simulink model "cruise_control"  (R2020b)
settings: Solver=VariableStepAuto  StartTime=0.0  StopTime=10.0  RelTol=1e-3
model workspace (MAT data in the model file):
  b = 50
  m = 1000
settings Model: DataDictionary=w2project3.sldd  Creator=rutvi  LastModifiedBy=rutvi
settings DataIOCC: SaveOutput=off  SaveTime=off

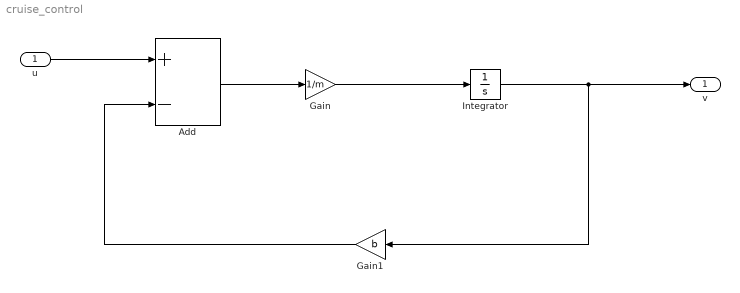
== system cruise_control ==
  u : Inport  OutDataTypeStr=double  PortDimensions=1
  Add : Sum  Inputs=+-
  Gain : Gain  Gain=1/m
  Gain1 : Gain  Gain=b
  Integrator : Integrator
  v : Outport  OutDataTypeStr=double  PortDimensions=1  SampleTime=0
  wires:
  u/1 -> Add/1
  Add/1 -> Gain/1
  Gain/1 -> Integrator/1
  Integrator/1 -> v/1, Gain1/1
  Gain1/1 -> Add/2
